simulink model "Openloop_Entrainment_I"  (R2015a)
settings: Solver=ode3  StartTime=0.0  StopTime=3000  FixedStep=0.01  RelTol=1e-5
values from neighbouring files (symbols this model uses):
  D = 1600/24    (= 66.6666666667)    [Openloop Entrainment.m]
  H0 = interp1q(Periodic_Solution(:,1),Periodic_Solution(:,4),time_shift(i))    [Openloop Entrainment.m]
  Imax = 1000    [Openloop Entrainment.m]
  n0 = interp1q(Periodic_Solution(:,1),Periodic_Solution(:,7),time_shift(i))    [Openloop Entrainment.m]
  Periodic_Solution = Periodic_Solution(Phase_Delay*100+1:end,:)    [Openloop Entrainment.m]
  Phase_Delay = 1    [Openloop Entrainment.m]
  T = 24    [Openloop Entrainment.m]
  tol = 0.01    [Openloop Entrainment.m]
  x0 = interp1q(Periodic_Solution(:,1),Periodic_Solution(:,2),time_shift(i))    [Openloop Entrainment.m]
  xc0 = interp1q(Periodic_Solution(:,1),Periodic_Solution(:,3),time_shift(i))    [Openloop Entrainment.m]
settings Model: Creator=Zhang Jiaxiang  LastModifiedBy=Jiawei Yin
settings DataIOCC: LimitDataPoints=off  SignalLoggingSaveFormat=ModelDataLogs
settings OptimizationCC: ExpressionDepthLimit=2147483647
settings DebuggingCC: UnderspecifiedInitializationDetection=Classic  MergeDetectMultiDrivingBlocksExec=none  FcnCallInpInsideContextMsg=UseLocalSettings  StateNameClashWarn=warning
settings GRTTargetCC: CombineOutputUpdateFcns=off  GRTInterface=on

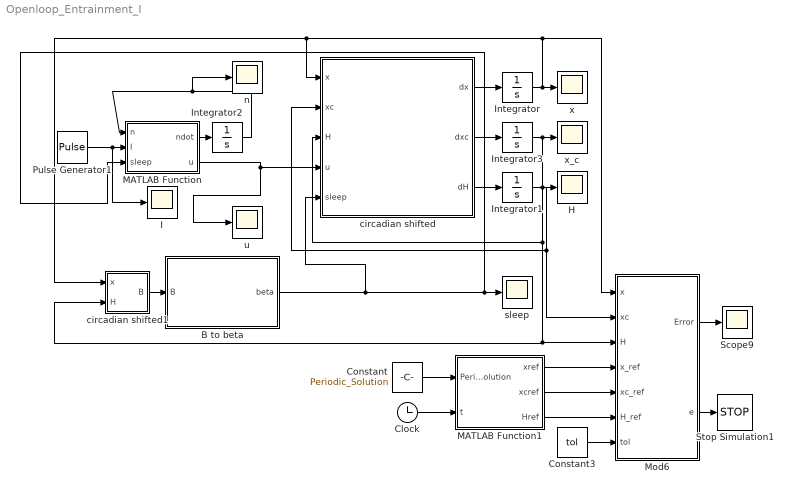
== system Openloop_Entrainment_I ==
  "B to beta " : Subsystem
  Clock : Clock
  Constant : Constant  Value=Periodic_Solution
  Constant3 : Constant  Value=tol
  H : Scope
      settings: TimeRange=auto  MaxDataPoints=1000000  SaveName=H  YMin=-0.03001  YMax=0.84118  SampleTime=-1  DataFormat=Array
  I : Scope
      settings: TimeRange=auto  MaxDataPoints=100000000  SaveName=I  YMin=-0.00064  YMax=0.00577  SampleTime=-1  DataFormat=Array
  Integrator : Integrator  InitialCondition=x0
  Integrator1 : Integrator  InitialCondition=H0
  Integrator2 : Integrator  InitialCondition=n0
  Integrator3 : Integrator  InitialCondition=xc0
  MATLAB Function : MATLAB Function  TreatAsAtomicUnit=on
      settings: PermitHierarchicalResolution=ParametersOnly
  MATLAB Function1 : MATLAB Function  TreatAsAtomicUnit=on
      settings: PermitHierarchicalResolution=ParametersOnly
  Mod6 : MATLAB Function  TreatAsAtomicUnit=on
      settings: PermitHierarchicalResolution=ParametersOnly
  Pulse Generator1 : DiscretePulseGenerator  PulseType=Time based  Amplitude=Imax  Period=T  PulseWidth=D  PhaseDelay=-Phase_Delay
  Scope9 : Scope
      settings: TimeRange=auto  LimitDataPoints=on  MaxDataPoints=5000  SaveToWorkspace=off  YMin=-10  YMax=10  SampleTime=-1  DataFormat=Array
  Stop Simulation1 : Stop
  circadian shifted : MATLAB Function  TreatAsAtomicUnit=on
      settings: PermitHierarchicalResolution=ParametersOnly
  circadian shifted1 : MATLAB Function  TreatAsAtomicUnit=on
      settings: PermitHierarchicalResolution=ParametersOnly
  n : Scope
      settings: TimeRange=auto  MaxDataPoints=1000000  SaveName=n  YMin=-0.03001  YMax=0.84118  SampleTime=-1  DataFormat=Array
  sleep : Scope
      settings: TimeRange=auto  MaxDataPoints=100000000  SaveName=sleep  YMin=-0.125  YMax=1.125  SampleTime=-1  DataFormat=Array
  u : Scope
      settings: TimeRange=auto  MaxDataPoints=1000000  SaveName=u  YMin=-0.03001  YMax=0.84118  SampleTime=-1  DataFormat=Array
  x : Scope
      settings: TimeRange=auto  MaxDataPoints=1000000  SaveName=x  YMin=-0.78539  YMax=7.06847  SampleTime=-1  DataFormat=Array
  x_c : Scope
      settings: TimeRange=auto  MaxDataPoints=1000000  SaveName=xc  YMin=-0.78539  YMax=7.06847  SampleTime=-1  DataFormat=Array
  wires:
  circadian shifted/1(dx) -> Integrator/1
  circadian shifted/3(dH) -> Integrator1/1
  Integrator1/1 -> circadian shifted1/2(H), Mod6/3(H), circadian shifted/3(H), H/1
  MATLAB Function/1(ndot) -> Integrator2/1
  Pulse Generator1/1 -> I/1, MATLAB Function/2(I)
  Integrator2/1 -> n/1, MATLAB Function/1(n)
  MATLAB Function/2(u) -> u/1, circadian shifted/4(u)
  circadian shifted1/1(B) -> "B to beta "/1(B)
  "B to beta "/1(beta) -> circadian shifted/5(sleep), MATLAB Function/3(sleep), sleep/1
  Integrator/1 -> Mod6/1(x), circadian shifted1/1(x), circadian shifted/1(x), x/1
  circadian shifted/2(dxc) -> Integrator3/1
  Integrator3/1 -> Mod6/2(xc), circadian shifted/2(xc), x_c/1
  Clock/1 -> MATLAB Function1/2(t)
  Constant/1 -> MATLAB Function1/1(Periodic_Solution)
  Mod6/2(e) -> Stop Simulation1/1
  Mod6/1(Error) -> Scope9/1
  Constant3/1 -> Mod6/7(tol)
  MATLAB Function1/1(xref) -> Mod6/4(x_ref)
  MATLAB Function1/2(xcref) -> Mod6/5(xc_ref)
  MATLAB Function1/3(Href) -> Mod6/6(H_ref)

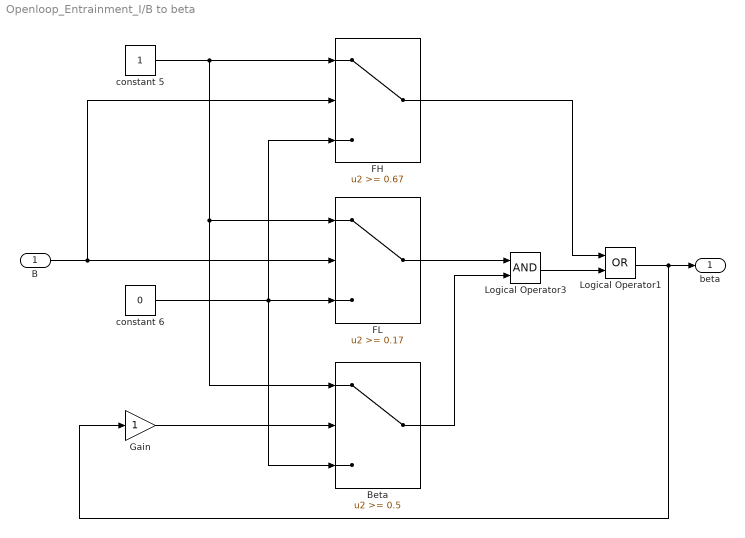
== system Openloop_Entrainment_I/B to beta  ==
  B : Inport
  Beta : Switch  Threshold=0.5
  FH : Switch  Threshold=0.67
  FL : Switch  Threshold=0.17
  Gain : Gain
  Logical Operator1 : Logic  Operator=OR  AllPortsSameDT=off  OutDataTypeStr=boolean
  Logical Operator3 : Logic  AllPortsSameDT=off  OutDataTypeStr=boolean
  constant 5 : Constant
  constant 6 : Constant  Value=0
  beta : Outport
  wires:
  constant 5/1 -> Beta/1, FL/1, FH/1
  constant 6/1 -> Beta/3, FH/3, FL/3
  B/1 -> FH/2, FL/2
  Logical Operator1/1 -> Gain/1, beta/1
  Gain/1 -> Beta/2
  FL/1 -> Logical Operator3/1
  Beta/1 -> Logical Operator3/2
  Logical Operator3/1 -> Logical Operator1/2
  FH/1 -> Logical Operator1/1

== matlab function Openloop_Entrainment_I/circadian shifted ==
  data: x input; xc input; H input; u input; dx output; dxc output; dH output; sleep input
function [ dx,dxc,dH] = fcn(x,xc,H,u,sleep)
%#eml
q = 1/3;
taux = 24.2;
k = 0.55;
mu=0.13;

B = u*(1-0.4*x)*(1-0.4*xc);
omega0=2*pi/24.2;
tr=18.2;
td=4.2;


dx = (pi/12)*(xc + B  + mu*(1/3*x + 4/3*x^3 - 256/105*x^7));
dxc = (pi/12)*(q*B *xc - (24/(taux*0.99729))^2*x - k*B*x);
dH=(1-H)*(1-sleep)/tr-H*sleep/td;

== matlab function Openloop_Entrainment_I/MATLAB Function ==
  data: n input; I input; ndot output; u output; sleep input
function [ndot,u] = fcn(n,I,sleep)
G=33.75;
alpha0=0.05;
beta=0.0075;
I0=9500;
alpha=alpha0*(I*(1-sleep)/I0)^0.5;
u=G*alpha*(1-n);
ndot=60*[alpha*(1-n)-beta*n];

== matlab function Openloop_Entrainment_I/MATLAB Function1 ==
  data: Periodic_Solution input; t input; xref output; xcref output; Href output
function [xref,xcref,Href] = fcn(Periodic_Solution,t)
xref=interp1q(Periodic_Solution(:,1),Periodic_Solution(:,2),t);
xcref=interp1q(Periodic_Solution(:,1),Periodic_Solution(:,3),t);
Href=interp1q(Periodic_Solution(:,1),Periodic_Solution(:,4),t);

== matlab function Openloop_Entrainment_I/circadian shifted1 ==
  data: x input; H input; B output
function B = fcn(x,H)
%#eml
B=H-0.1333*x;

== matlab function Openloop_Entrainment_I/Mod6 ==
  data: Error output; x input; xc input; H input; x_ref input; xc_ref input; e output; H_ref input; tol input
function [Error,e] = fcn(x,xc,H,x_ref,xc_ref,H_ref,tol)
%#codegen
Error=(H-H_ref)^2+(x-x_ref)^2+(xc-xc_ref)^2;
e=Error<tol;
